simulink model "sixpulseconv"  (R2020b)
settings: Solver=VariableStepAuto  StartTime=0.0  StopTime=0.06  RelTol=1e-3
libraries: powerlib x13, powerlib_meascontrol x1
settings Model: Creator=Anuj Attri  LastModifiedBy=Anuj Attri

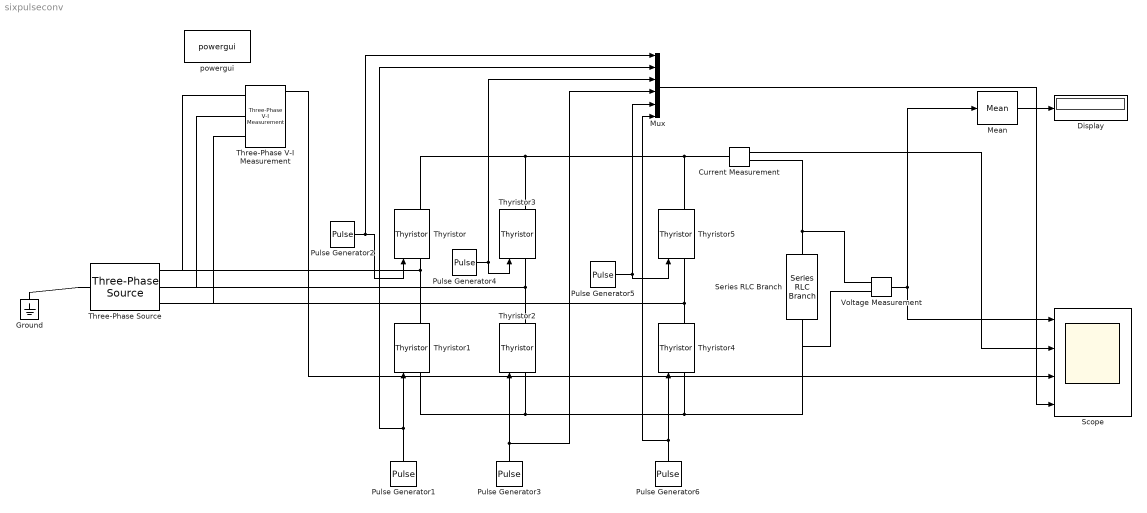
== system sixpulseconv ==
  Current Measurement : powerlib/Measurements/Current Measurement  PhasorSimulation=off  OutputType=Complex  PSBequivalent=0
  Display : Display
  Ground : powerlib/Elements/Ground  LConnTagsString=a
  Mean : powerlib_meascontrol/Measurements/Mean  Freq=50  Vinit=0  Ts=0
  Mux : Mux  Inputs=6
  Pulse Generator1 : DiscretePulseGenerator  PulseType=Time based  Period=0.02  PulseWidth=5  PhaseDelay=11.667e-3
  Pulse Generator2 : DiscretePulseGenerator  PulseType=Time based  Period=0.02  PulseWidth=5  PhaseDelay=1.667e-3
  Pulse Generator3 : DiscretePulseGenerator  PulseType=Time based  Period=0.02  PulseWidth=5  PhaseDelay=18.333e-3
  Pulse Generator4 : DiscretePulseGenerator  PulseType=Time based  Period=0.02  PulseWidth=5  PhaseDelay=8.33e-3
  Pulse Generator5 : DiscretePulseGenerator  PulseType=Time based  Period=0.02  PulseWidth=5  PhaseDelay=15e-3
  Pulse Generator6 : DiscretePulseGenerator  PulseType=Time based  Period=0.02  PulseWidth=5  PhaseDelay=5e-3
  Scope : Scope  NumInputPorts=4
  Series RLC Branch : powerlib/Elements/Series RLC Branch  LConnTagsString=__new0  RConnTagsString=__new0  BranchType=R  Resistance=10  Inductance=10e-3  SetiL0=off  InitialCurrent=0  Capacitance=1e-6  Setx0=off  InitialVoltage=0  Measurements=None
  Three-Phase V-I Measurement : powerlib/Measurements/Three-Phase V-I Measurement  VoltageMeasurement=phase-to-ground  SetLabelV=off  LabelV=Vabc  Vpu=off  VpuLL=off  CurrentMeasurement=yes  SetLabelI=off  LabelI=Iabc  Ipu=off  Pbase=100e6  Vbase=500e3  OutputType=Complex  PhasorSimulation=off  PSBequivalent=0
  Three-Phase Source : powerlib/Electrical Sources/Three-Phase Source  InternalConnection=Yn  VoltagePhases=off  Voltage=415  PhaseAngle=0  Voltage_phases=[25e3 25e3 25e3]/sqrt(3)  PhaseAngles_phases=[0 -120 +120]  Frequency=50  NonIdealSource=off  SpecifyImpedance=off  Resistance=0.8929  Inductance=16.58e-3  ShortCircuitLevel=100e6  BaseVoltage=25e3  XRratio=7  BusType=swing  Pref=10e3  Qref=0  Prefabc=[10e3, 10e3, 10e3]  Qrefabc=[0, 0, 0]  Qmin=-inf  Qmax=inf
  Thyristor{,1..5} (6 alike) : powerlib/Power Electronics/Thyristor  Ron=0.001  Lon=0  Vf=0.8  IC=0  Rs=500  Cs=250e-9  Measurements=on
  Voltage Measurement : powerlib/Measurements/Voltage Measurement  PhasorSimulation=off  OutputType=Complex  PSBequivalent=0
  powergui : powerlib/powergui  Priority=1  SimulationMode=Continuous  SampleTime=50e-6  frequency=60  Iterations=50  frequencyindice=50  Pbase=100e6  ErrMax=1e-4  UnitsV=kV  UnitsW=MW  buscounter=0  FunctionMessages=off  echomessages=off  EnableUseOfTLC=off  CurrentSourceSwitches=off  DisableSnubberDevices=off  DisableRonSwitches=off  DisableVfSwitches=off  DisplayEquations=off  AutomaticDiscreteSolvers=off  SolverType=Tustin/Backward Euler (TBE)  Interpol=off  ExternalGateDelay=off  methode=off  Ts=100  x0status=blocks  SPID=on  SwTol=0  HookPort=off  NonlinearTolerance=1e-4  nMaxIteration=100  ContinueOnMaxIteration=off  RestoreLinks=warning  ResistiveCurrentMeasurement=off  Frange=[0:2:500]  Ylog=off  Xlog=on  ShowGrid=off  save=off  variable=ZData  structure=0  ZoomFFT=off  StartTime=0.0  cycles=1  DisplayStyle=1  fundamental=60  FreqAxis=off  MaxFrequency=1000  frequencyindicesteady=1  RmsSteady=1  display=off
  wires:
  Voltage Measurement/1 -> Mean/1, Scope/1
  Mean/1 -> Display/1
  Pulse Generator2/1 -> Mux/1, Thyristor/1
  Pulse Generator1/1 -> Mux/2, Thyristor1/1
  Pulse Generator3/1 -> Mux/4, Thyristor2/1
  Pulse Generator4/1 -> Mux/3, Thyristor3/1
  Pulse Generator5/1 -> Thyristor5/1, Mux/5
  Pulse Generator6/1 -> Mux/6, Thyristor4/1
  Current Measurement/1 -> Scope/2
  Three-Phase V-I Measurement/1 -> Scope/3
  Mux/1 -> Scope/4
  connections:
  Thyristor/RConn1 -- Thyristor3/RConn1 -- Thyristor5/RConn1 -- Current Measurement/LConn1
  Thyristor/LConn1 -- Three-Phase V-I Measurement/LConn1 -- Three-Phase Source/RConn1 -- Thyristor1/RConn1
  Thyristor1/LConn1 -- Thyristor2/LConn1 -- Voltage Measurement/LConn2 -- Series RLC Branch/RConn1 -- Thyristor4/LConn1
  Thyristor3/LConn1 -- Three-Phase V-I Measurement/LConn2 -- Three-Phase Source/RConn2 -- Thyristor2/RConn1
  Thyristor5/LConn1 -- Three-Phase V-I Measurement/LConn3 -- Three-Phase Source/RConn3 -- Thyristor4/RConn1
  Current Measurement/RConn1 -- Voltage Measurement/LConn1 -- Series RLC Branch/LConn1
  Three-Phase Source/LConn1 -- Ground/LConn1
